simulink model "engine_core"  (R2026a)
settings: Solver=VariableStepAuto  StopTime=300
undefined symbols (not defined in the file): engine

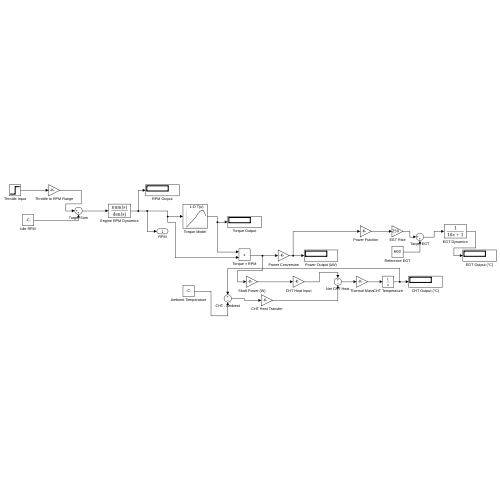
[thumbnail: Simulink's stored preview of the top-level diagram]
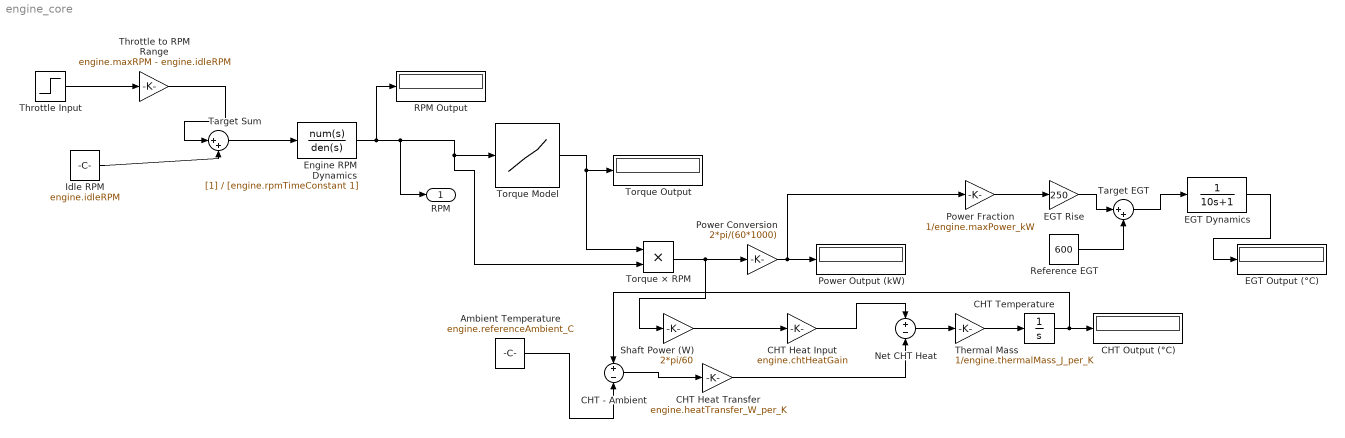
== system engine_core ==
  Ambient Temperature : Constant  Value=engine.referenceAmbient_C
  CHT - Ambient : Sum  Inputs=+-
  CHT Heat Input : Gain  Gain=engine.chtHeatGain
  CHT Heat Transfer : Gain  Gain=engine.heatTransfer_W_per_K
  CHT Output (°C) : Display
  CHT Temperature : Integrator  InitialCondition=engine.referenceAmbient_C
  EGT Dynamics : TransferFcn  Denominator=[10 1]
  EGT Output (°C) : Display
  EGT Rise : Gain  Gain=250
  Engine RPM Dynamics : TransferFcn  Denominator=[engine.rpmTimeConstant 1]
  Idle RPM : Constant  Value=engine.idleRPM
  Net CHT Heat : Sum  Inputs=+-
  Power Conversion : Gain  Gain=2*pi/(60*1000)
  Power Fraction : Gain  Gain=1/engine.maxPower_kW
  Power Output (kW) : Display
  RPM Output : Display
  Reference EGT : Constant  Value=600
  Shaft Power (W) : Gain  Gain=2*pi/60
  Target EGT : Sum  Inputs=|++
  Target Sum : Sum  Inputs=|++
  Thermal Mass : Gain  Gain=1/engine.thermalMass_J_per_K
  Throttle Input : Step  Time=0  FinalValue=0.9  SampleTime=0
  Throttle to RPM Range : Gain  Gain=engine.maxRPM - engine.idleRPM
  "Torque Model " : Lookup_n-D  NumberOfTableDimensions=1  BreakpointsForDimension1=[1500 2500 3500 4000 4500 4900 5200 5500 5800]  Table=[90 105 120 132 140 144 142 135 126]  InternalRulePriority=Speed  RndMeth=Simplest
  Torque Output : Display
  Torque × RPM : Product
  RPM : Outport
  wires:
  Throttle Input/1 -> Throttle to RPM Range/1
  Throttle to RPM Range/1 -> Target Sum/1
  Idle RPM/1 -> Target Sum/2
  Target Sum/1 -> Engine RPM Dynamics/1
  Engine RPM Dynamics/1 -> RPM/1, Torque × RPM/2, "Torque Model "/1, RPM Output/1
  "Torque Model "/1 -> Torque × RPM/1, Torque Output/1
  Torque × RPM/1 -> Power Conversion/1, Shaft Power (W)/1
  Power Conversion/1 -> Power Fraction/1, Power Output (kW)/1
  Shaft Power (W)/1 -> CHT Heat Input/1
  CHT Heat Input/1 -> Net CHT Heat/1
  Net CHT Heat/1 -> Thermal Mass/1
  Thermal Mass/1 -> CHT Temperature/1
  CHT Temperature/1 -> CHT Output (°C)/1, CHT - Ambient/1
  Ambient Temperature/1 -> CHT - Ambient/2
  CHT - Ambient/1 -> CHT Heat Transfer/1
  CHT Heat Transfer/1 -> Net CHT Heat/2
  Power Fraction/1 -> EGT Rise/1
  EGT Rise/1 -> Target EGT/1
  Reference EGT/1 -> Target EGT/2
  Target EGT/1 -> EGT Dynamics/1
  EGT Dynamics/1 -> EGT Output (°C)/1
